simulink model "a1_Conventional_IFPR_EUROPE_10s_C"  (R2019a)
settings: Solver=VariableStepAuto  StartTime=0  StopTime=80  RelTol=1e-3
values from neighbouring files (symbols this model uses):
  E_load = 150    [a1_Conventional_mechlimit_EUR.m]    (also in calc_criticaltime.m; calc_nadir_IBFPR_SI.m; calc_variables_a1Ta.m; power_reserve.m)
  H = Ek/Sb    (= 0.375)    [a1_Conventional_mechlimit_EUR.m]    (also in calc_criticaltime.m = 3.75; calc_nadir_IBFPR_SI.m = 1.035; calc_variables_a1Ta.m = 2.25; power_reserve.m = 3.75)
  Sb = 200    [a1_Conventional_mechlimit_EUR.m]    (also in calc_criticaltime.m; calc_nadir_IBFPR_SI.m = 166.666666667; calc_variables_a1Ta.m = 166.666666667; power_reserve.m)
  T_1 = data1(2)    [a1_Conventional_mechlimit_EUR.m]    (also in calc_criticaltime.m; calc_nadir_IBFPR_SI.m; calc_variables_a1Ta.m; power_reserve.m)
  T_2 = data1(3)    [a1_Conventional_mechlimit_EUR.m]    (also in calc_criticaltime.m; calc_nadir_IBFPR_SI.m; calc_variables_a1Ta.m; power_reserve.m)
  T_3 = data1(4)    [a1_Conventional_mechlimit_EUR.m]    (also in calc_criticaltime.m; calc_nadir_IBFPR_SI.m; calc_variables_a1Ta.m; power_reserve.m)
  T_4 = data1(5)    [a1_Conventional_mechlimit_EUR.m]    (also in calc_criticaltime.m; calc_nadir_IBFPR_SI.m; calc_variables_a1Ta.m; power_reserve.m)
  un = 0.02    [calc_nadir_IBFPR_SI.m]    (also in calc_variables_a1Ta.m)
settings Model: Creator=estuser04  LastModifiedBy=Alejandro
settings SolverCC: AlgebraicLoopSolver=LineSearch
settings DataIOCC: ReturnWorkspaceOutputs=off
settings DebuggingCC: ArithmeticOperatorsInVariantConditions=warning

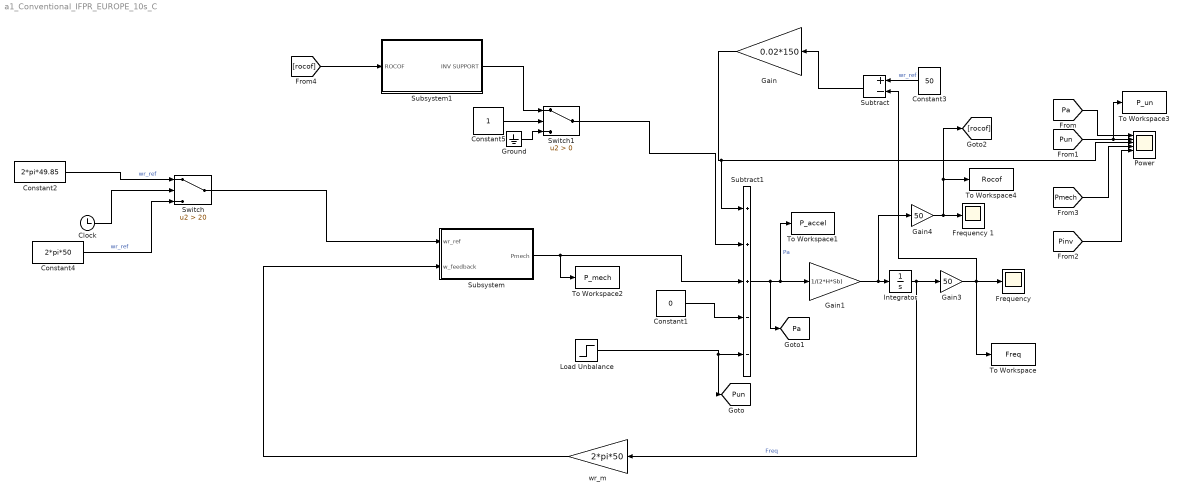
== system a1_Conventional_IFPR_EUROPE_10s_C ==
  Clock : Clock
  Constant1 : Constant  Value=0
  Constant2 : Constant  Value=2*pi*49.85
  Constant3 : Constant  Value=50
  Constant4 : Constant  Value=2*pi*50
  Constant5 : Constant
  "Frequency " : Scope
  Frequency 1 : Scope
  Gain : Gain  Gain=0.02*150
  Gain1 : Gain  Gain=1/(2*H*Sb)
  Gain3 : Gain  Gain=50
  Gain4 : Gain  Gain=50
  Ground : Ground
  Integrator : Integrator  InitialCondition=1
  Load Unbalance : Step  Time=0  After=E_load*un  SampleTime=0
  Power : Scope  NumInputPorts=6
  Subsystem : Subsystem
  Subsystem1 : Subsystem
  Subtract : Sum  Inputs=+-
  Subtract1 : Sum  Inputs=+++--
  Switch : Switch  Criteria=u2 > Threshold  Threshold=20
  Switch1 : Switch  Criteria=u2 > Threshold
  To Workspace : ToWorkspace  VariableName=Freq  SaveFormat=Timeseries  SampleTime=-1
  To Workspace1 : ToWorkspace  VariableName=P_accel  SaveFormat=Timeseries  SampleTime=-1
  To Workspace2 : ToWorkspace  VariableName=P_mech  SaveFormat=Timeseries  SampleTime=-1
  To Workspace3 : ToWorkspace  VariableName=P_un  SaveFormat=Timeseries  SampleTime=-1
  To Workspace4 : ToWorkspace  VariableName=Rocof  SaveFormat=Timeseries  SampleTime=-1
  "wr_m " : Gain  Gain=2*pi*50
  tag scope: Pa=global, Pun=global
  wires:
  Integrator/1 -> Gain3/1, "wr_m "/1  "Freq"
  Subtract1/1 -> [Pa], To Workspace1/1, Gain1/1  "Pa"
  Constant1/1 -> Subtract1/4
  Constant2/1 -> Switch/1  "wr_ref"
  "wr_m "/1 -> Subsystem/2(w_feedback)
  Subsystem/1(Pmech) -> Subtract1/3, To Workspace2/1
  [Pa] -> Power/1
  [Pun] -> To Workspace3/1, Power/2
  [Pmech] -> Power/4
  Gain1/1 -> Gain4/1, Integrator/1
  Gain4/1 -> [rocof], To Workspace4/1, Frequency 1/1
  Constant3/1 -> Subtract/1  "wr_ref"
  Subtract/1 -> Gain/1
  Gain3/1 -> Subtract/2, To Workspace/1, "Frequency "/1
  Gain/1 -> Subtract1/1, Power/3
  Load Unbalance/1 -> Subtract1/5, [Pun]
  Constant4/1 -> Switch/3  "wr_ref"
  Clock/1 -> Switch/2
  Switch/1 -> Subsystem/1(wr_ref)
  [Pinv] -> Power/5
  Subsystem1/1(INV SUPPORT) -> Switch1/1
  Ground/1 -> Switch1/3
  Constant5/1 -> Switch1/2
  Switch1/1 -> Subtract1/2
  [rocof] -> Subsystem1/1(ROCOF)

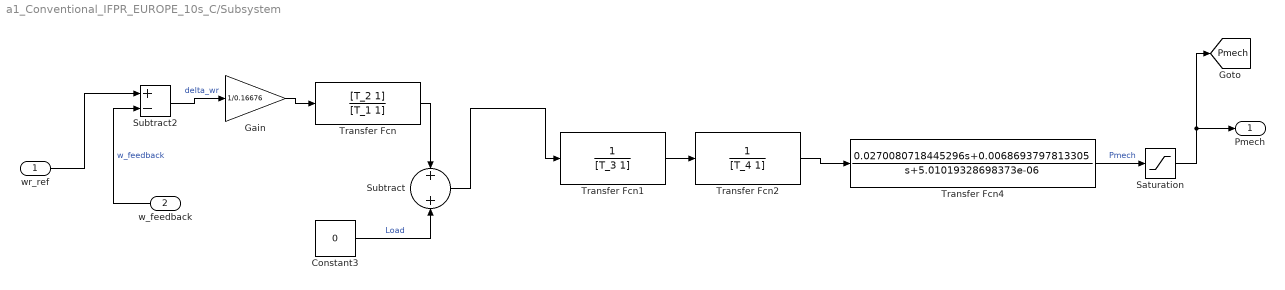
== system a1_Conventional_IFPR_EUROPE_10s_C/Subsystem ==
  wr_ref : Inport
  w_feedback : Inport  Port=2
  Constant3 : Constant  Value=0
  Gain : Gain  Gain=1/0.16676
  Saturation : Saturate  UpperLimit=un*E_load  LowerLimit=0
  Subtract : Sum
  Subtract2 : Sum  Inputs=+-
  Transfer Fcn : TransferFcn  Numerator=[T_2 1]  Denominator=[T_1 1]
  Transfer Fcn1 : TransferFcn  Denominator=[T_3 1]
  Transfer Fcn2 : TransferFcn  Denominator=[T_4 1]
  Transfer Fcn4 : TransferFcn  Numerator=[0.0270080718445296 0.0068693797813305]  Denominator=[1 5.01019328698373e-06]
  Pmech : Outport
  tag scope: Pmech=global
  wires:
  Constant3/1 -> Subtract/2  "Load"
  Transfer Fcn/1 -> Subtract/1
  Gain/1 -> Transfer Fcn/1
  Transfer Fcn2/1 -> Transfer Fcn4/1
  w_feedback/1 -> Subtract2/2  "w_feedback"
  Transfer Fcn1/1 -> Transfer Fcn2/1
  wr_ref/1 -> Subtract2/1
  Transfer Fcn4/1 -> Saturation/1  "Pmech"
  Subtract2/1 -> Gain/1  "delta_wr"
  Subtract/1 -> Transfer Fcn1/1
  Saturation/1 -> [Pmech], Pmech/1

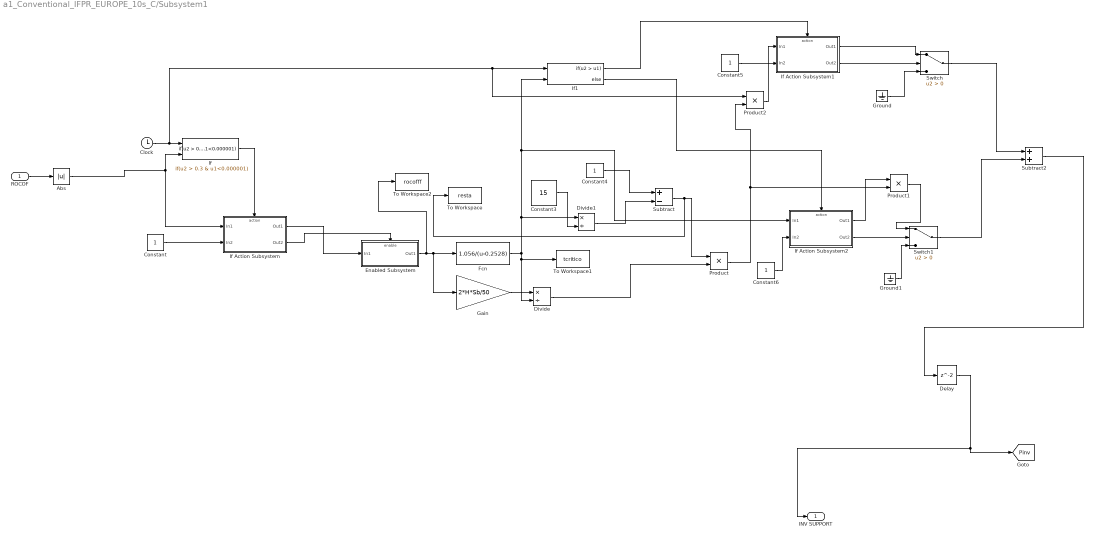
== system a1_Conventional_IFPR_EUROPE_10s_C/Subsystem1 ==
  ROCOF : Inport
  Abs : Abs
  Clock : Clock
  Constant{,4..6} (4 alike) : Constant
  Constant3 : Constant  Value=15
  Delay : Delay  SampleTime=0.001
  Divide : Product  Inputs=*/
  Divide1 : Product  Inputs=*/
  Enabled Subsystem : Subsystem  TreatAsAtomicUnit=on
  Fcn : Fcn  Expr=1.056/(u-0.2528)
  Gain : Gain  Gain=2*H*Sb/50
  Ground : Ground
  Ground1 : Ground
  If : If  NumInputs=2  IfExpression=u2 > 0.3 & u1<0.000001  ShowElse=off
  If Action Subsystem : Subsystem  TreatAsAtomicUnit=on
  If Action Subsystem1 : Subsystem  TreatAsAtomicUnit=on
  If Action Subsystem2 : Subsystem  TreatAsAtomicUnit=on
  If1 : If  NumInputs=2  IfExpression=u2 > u1
  Product : Product
  Product1 : Product
  Product2 : Product
  Subtract : Sum  Inputs=+-
  Subtract2 : Sum
  Switch : Switch  Criteria=u2 > Threshold
  Switch1 : Switch  Criteria=u2 > Threshold
  To Workspace : ToWorkspace  VariableName=resta  SaveFormat=Timeseries  SampleTime=-1
  To Workspace1 : ToWorkspace  VariableName=tcritico  SaveFormat=Timeseries  SampleTime=-1
  To Workspace2 : ToWorkspace  VariableName=rocofff  SaveFormat=Timeseries  SampleTime=-1
  INV SUPPORT : Outport
  tag scope: Pinv=global
  wires:
  Switch1/1 -> Subtract2/2
  If Action Subsystem2/2(Out2) -> Switch1/2
  Divide/1 -> Product/2
  Product/1 -> Product1/2, Product2/2
  Constant4/1 -> Subtract/1
  Fcn/1 -> Divide/2, To Workspace1/1, If Action Subsystem2/1(In1), If1/2, Divide1/1
  If Action Subsystem/2(Out2) -> Enabled Subsystem/Enable
  Clock/1 -> Product2/1, If1/1, If/1
  Ground/1 -> Switch/3
  Divide1/1 -> Subtract/2
  Constant3/1 -> Divide1/2
  Enabled Subsystem/1(Out1) -> To Workspace2/1, Gain/1, Fcn/1
  If Action Subsystem/1(Out1) -> Enabled Subsystem/1(In1)
  Subtract/1 -> To Workspace/1, Product/1
  If Action Subsystem1/2(Out2) -> Switch/2
  If1/1 -> If Action Subsystem1/Action
  Subtract2/1 -> Delay/1
  Gain/1 -> Divide/1
  Ground1/1 -> Switch1/3
  If Action Subsystem2/1(Out1) -> Product1/1
  ROCOF/1 -> Abs/1
  Product1/1 -> Switch1/1
  If Action Subsystem1/1(Out1) -> Switch/1
  Constant6/1 -> If Action Subsystem2/2(In2)
  Constant5/1 -> If Action Subsystem1/2(In2)
  Switch/1 -> Subtract2/1
  Constant/1 -> If Action Subsystem/2(In2)
  Abs/1 -> If Action Subsystem/1(In1), If/2
  If1/2 -> If Action Subsystem2/Action
  Product2/1 -> If Action Subsystem1/1(In1)
  Delay/1 -> [Pinv], INV SUPPORT/1
  If/1 -> If Action Subsystem/Action

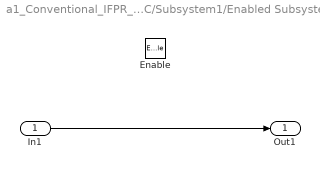
== system a1_Conventional_IFPR_EUROPE_10s_C/Subsystem1/Enabled Subsystem ==
  In1 : Inport
  Enable : EnablePort
  Out1 : Outport  InitialOutput=0.0000000000000000001
  wires:
  In1/1 -> Out1/1

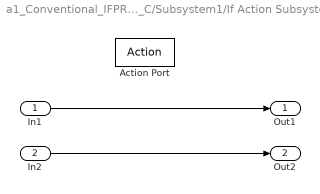
== system a1_Conventional_IFPR_EUROPE_10s_C/Subsystem1/If Action Subsystem ==
  In1 : Inport
  In2 : Inport  Port=2
  Action Port : ActionPort  ActionPortLabel=if(u2 > 0.3 & u1<0.000001)
  Out1 : Outport  InitialOutput=0
  Out2 : Outport  Port=2  InitialOutput=0
  wires:
  In1/1 -> Out1/1
  In2/1 -> Out2/1

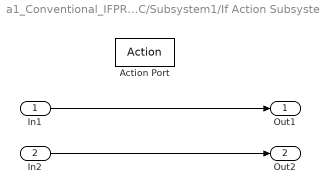
== system a1_Conventional_IFPR_EUROPE_10s_C/Subsystem1/If Action Subsystem1 ==
  In1 : Inport
  In2 : Inport  Port=2
  Action Port : ActionPort  ActionPortLabel=if(u2 > u1)
  Out1 : Outport  OutputWhenDisabled=reset  InitialOutput=0
  Out2 : Outport  Port=2  OutputWhenDisabled=reset  InitialOutput=0
  wires:
  In1/1 -> Out1/1
  In2/1 -> Out2/1

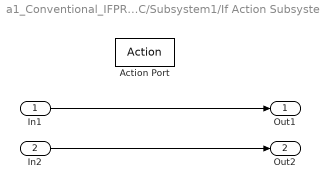
== system a1_Conventional_IFPR_EUROPE_10s_C/Subsystem1/If Action Subsystem2 ==
  In1 : Inport
  In2 : Inport  Port=2
  Action Port : ActionPort  ActionPortLabel=else
  Out1 : Outport  OutputWhenDisabled=reset  InitialOutput=0
  Out2 : Outport  Port=2  InitialOutput=0
  wires:
  In1/1 -> Out1/1
  In2/1 -> Out2/1
